simulink model "Mining_data"  (R2019b)
settings: Solver=VariableStepAuto  StartTime=0.0  StopTime=7  FixedStep=20e-3  MaxStep=20e-3  RelTol=1e-3
undefined symbols (not defined in the file or in its folder): sigbuilder_block
libraries: lib_robotinohardware x5
settings Model: EnablePacing=on  Creator=indorewala  LastModifiedBy=Олег
settings DataIOCC: LimitDataPoints=on  SaveFormat=Array  SignalLoggingSaveFormat=ModelDataLogs  ReturnWorkspaceOutputs=off
settings OptimizationCC: ExpressionDepthLimit=2147483647  InitFltsAndDblsToZero=on  LifeSpan=inf
settings DebuggingCC: UnderspecifiedInitializationDetection=Classic  MergeDetectMultiDrivingBlocksExec=none  SolverPrmCheckMsg=warning  FcnCallInpInsideContextMsg=warning  StateNameClashWarn=warning  SFUnexpectedBacktrackingDiag=warning  SFNoUnconditionalDefaultTransitionDiag=warning  SFExecutionAtInitializationDiag=none  ArithmeticOperatorsInVariantConditions=warning
settings HardwareCC: ProdBitPerPointer=32  ProdBitPerSizeT=32  ProdBitPerPtrDiffT=32  ProdLargestAtomicFloat=None  ProdIntDivRoundTo=Undefined  ProdEndianess=Unspecified  ProdWordSize=32  ProdHWDeviceType=32-bit Generic
settings ModelReferenceCC: PropagateSignalLabelsOutOfModel=off
settings SFSimCC: SimUseLocalCustomCode=off  CustomCodeUndefinedFunction=UseInterfaceOnly
settings RTWCC: RTWUseLocalCustomCode=off
settings CodeAppCC: StateflowObjectComments=on
settings GRTTargetCC: TargetLangStandard=C89/C90 (ANSI)  CombineOutputUpdateFcns=off  GRTInterface=on
settings ConfigComp: CovMetricSettings=dw  CovHtmlReporting=on  CovSaveCumulativeToWorkspaceVar=on  CovSaveSingleToWorkspaceVar=on  CovExternalEMLEnable=off

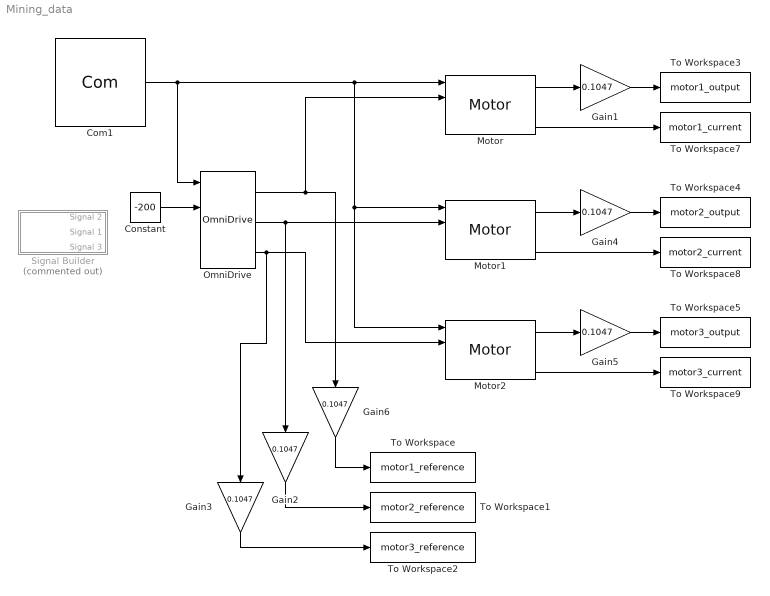
== system Mining_data ==
  Com1 : lib_robotinohardware/Com  ip='172.26.1.0'
  Constant : Constant  Value=-200
  Gain{1..6} (6 alike) : Gain  Gain=0.1047
  Motor : lib_robotinohardware/Motor  num=0  kp=200  ki=10  kd=0
  Motor1 : lib_robotinohardware/Motor  num=1  kp=200  ki=10  kd=0
  Motor2 : lib_robotinohardware/Motor  num=2  kp=200  ki=10  kd=0
  OmniDrive : lib_robotinohardware/OmniDrive
  Signal Builder : Subsystem  Tag=STV Subsys  Commented=on  LoadFcn=sigbuilder_block('load');  StartFcn=sigbuilder_block('start');  StopFcn=sigbuilder_block('stop');  ClipboardFcn=sigbuilder_block('clipboard');  mask(Sigbuilder block){tuvar=[0:10]}
      mask help: Simulink:masks:SigbuilderBlock_MD
      mask init:
      | if ~strcmp(get_param(bdroot(gcbh),'SimulationStatus'),'stopped') tuvar = sigbuilder_block('maskInit'); end
      settings: CopyFcn=sigbuilder_block('copy');  DeleteFcn=sigbuilder_block('delete');  ModelCloseFcn=sigbuilder_block('modelClose');  PreSaveFcn=sigbuilder_block('preSave');  PauseFcn=sigbuilder_block('pause');  ContinueFcn=sigbuilder_block('continue');  NameChangeFcn=sigbuilder_block('namechange');  OpenFcn=sigbuilder_block('open',[5.4 30 1141.2 522.6 ]);  CloseFcn=sigbuilder_block('close');
      mask Display: plot(0, 0, 100, 100,[2, 2, 32, 32, 2], [68, 8, 8, 68, 68],[32, 2], [38, 38], [32, 19, 2],[53, 60, 44], [32, 17, 17, 2],[16, 16, 31, 31]);txt = getActiveGroup(gcbh);text(2, 100, txt,'verticalAlignment', 'top');
  To Workspace : ToWorkspace  VariableName=motor1_reference  SaveFormat=Timeseries  SampleTime=-1
  To Workspace1 : ToWorkspace  VariableName=motor2_reference  SaveFormat=Timeseries  SampleTime=-1
  To Workspace2 : ToWorkspace  VariableName=motor3_reference  SaveFormat=Timeseries  SampleTime=-1
  To Workspace3 : ToWorkspace  VariableName=motor1_output  SaveFormat=Timeseries  SampleTime=-1
  To Workspace4 : ToWorkspace  VariableName=motor2_output  SaveFormat=Timeseries  SampleTime=-1
  To Workspace5 : ToWorkspace  VariableName=motor3_output  SaveFormat=Timeseries  SampleTime=-1
  To Workspace7 : ToWorkspace  VariableName=motor1_current  SaveFormat=Timeseries  SampleTime=-1
  To Workspace8 : ToWorkspace  VariableName=motor2_current  SaveFormat=Timeseries  SampleTime=-1
  To Workspace9 : ToWorkspace  VariableName=motor3_current  SaveFormat=Timeseries  SampleTime=-1
  wires:
  Com1/1 -> OmniDrive/1, Motor/1, Motor2/1, Motor1/1
  Motor/1 -> Gain1/1
  OmniDrive/1 -> Gain6/1, Motor/2
  OmniDrive/2 -> Gain2/1, Motor1/2
  OmniDrive/3 -> Gain3/1, Motor2/2
  Motor1/1 -> Gain4/1
  Motor2/1 -> Gain5/1
  Gain6/1 -> To Workspace/1
  Gain2/1 -> To Workspace1/1
  Gain3/1 -> To Workspace2/1
  Gain1/1 -> To Workspace3/1
  Gain4/1 -> To Workspace4/1
  Gain5/1 -> To Workspace5/1
  Motor/3 -> To Workspace7/1
  Motor1/3 -> To Workspace8/1
  Motor2/3 -> To Workspace9/1
  Constant/1 -> OmniDrive/2

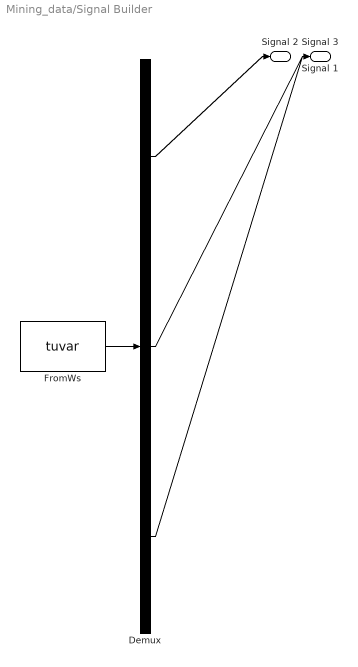
== system Mining_data/Signal Builder ==
  Demux : Demux  Tag=STV Demux  Outputs=3
  FromWs : FromWorkspace  Tag=STV FromWs  VariableName=tuvar  SampleTime=0
      SigBuilderData=|
      | common.afterFinalStr = 'Extrapolate'
      | common.sampleTime = 0
      | dataSet.timeRange = [0 180]
      | dataSet.name = 'Group 1'
      | sbobj.Groups.Name = 'Group 1'
      | sbobj.Groups.Signals(1).Name = 'Signal 2'
      | sbobj.Groups.Signals(1).XData = [0 1 1 7.4 7.4 9.6 9.6 13.6 13.6 20 20 26 26 30.8 30.8 35.8 35.8 40 40 43.8 43.8 48.2 48.2 57.4 57.4 180]
      | sbobj.Groups.Signals(1).YData = [0 0 100 100 0 0 -300 -300 0 0 200 200 0 0 -200 -200 0 0 300 300 0 0 -100 -100 0 0]
      | sbobj.Groups.Signals(2).Name = 'Signal 1'
      | sbobj.Groups.Signals(2).XData = [0 8.57142857143 59.2 59.2 66.4 66.4 70.6 70.6 74.6 74.6 81.4 81.4 88.6 88.6 93.4 93.4 99.4 99.4 103.6 103.6 107.8 107.8 111.6 111.6 119 119 180]
      | sbobj.Groups.Signals(2).YData = [0 0 0 100 100 0 0 -300 -300 0 0 200 200 0 0 -200 -200 0 0 300 300 0 0 -100 -100 0 0]
      | sbobj.Groups.Signals(3).Name = 'Signal 3'
      | sbobj.Groups.Signals(3).XData = [0 8.57142857143 123 123 131.6 131.6 134.8 134.8 140 140 143.4 143.4 148.6 148.6 153 153 159.2 159.2 163 163 168.6 168.6 171.6 171.6 179 179 180]
      | sbobj.Groups.Signals(3).YData = [0 0 0 20 20 0 0 -40 -40 0 0 30 30 0 0 -30 -30 0 0 40 40 0 0 -20 -20 0 0]
      | sbobj.Groups.TimeRange = [0 180]
  Signal 2 : Outport  Tag=STV Outport
  Signal 1 : Outport  Tag=STV Outport  Port=2
  Signal 3 : Outport  Tag=STV Outport  Port=3
  wires:
  FromWs/1 -> Demux/1
  Demux/1 -> Signal 2/1
  Demux/2 -> Signal 1/1
  Demux/3 -> Signal 3/1
